simulink model "Arm_core_design_block"  (R2021a)
settings: Solver=VariableStepAuto  StartTime=0.0  StopTime=500  RelTol=1e-3
undefined symbols (not defined in the file or in its folder): AXI4, Lite
libraries: hdlBasic x907, xbsIndex_r4 x1
(part 7 of 7)

== system Arm_core_design_block/rotation9/Subsystem9 ==
  rst : Inport
  reg_i : Inport  Port=2
  Absolute1 : hdlBasic/Absolute  precision=User Defined  arith_type="Signed  (2's comp)"  n_bits=16  bin_pt=13  quantization=Truncate  overflow=Saturate  en=off  latency=0  XmcBlockStatus=1  maskContainerNames=tabcontainer1  block_type=abs  block_config=sysgen:Abs_config
  Accumulator1 : hdlBasic/Accumulator  operation=Add  n_bits=16  overflow=Wrap  scale=1  rst=on  hasbypass=off  en=on  latency=1  msb_inp=100  msb=100  lsb=-100  use_behavioral_HDL=on  implementation=Fabric  XmcBlockStatus=1  maskContainerNames=group3  block_type=accum  block_config=sysgen:Accum_config
  Constant4 : hdlBasic/Constant  const=0.019  gui_display_data_type=Fixed-point  arith_type=Signed (2's comp)  n_bits=16  bin_pt=14  preci_type=Single  exp_width=8  frac_width=24  explicit_period=off  period=1  XmcBlockStatus=1  maskContainerNames=tabcontainer1  block_type=constant  block_config=sysgen:Constant_config
  Constant5 : hdlBasic/Constant  const=1  gui_display_data_type=Fixed-point  arith_type=Unsigned  n_bits=16  bin_pt=1  preci_type=Single  exp_width=8  frac_width=24  explicit_period=off  period=1  XmcBlockStatus=1  maskContainerNames=tabcontainer1  block_type=constant  block_config=sysgen:Constant_config
  Constant6 : hdlBasic/Constant  const=3  gui_display_data_type=Fixed-point  arith_type=Unsigned  n_bits=16  bin_pt=1  preci_type=Single  exp_width=8  frac_width=24  explicit_period=off  period=1  XmcBlockStatus=1  maskContainerNames=tabcontainer1  block_type=constant  block_config=sysgen:Constant_config
  Constant7 : hdlBasic/Constant  const=0  gui_display_data_type=Boolean  arith_type=Boolean  n_bits=16  bin_pt=1  preci_type=Single  exp_width=8  frac_width=24  explicit_period=off  period=1  XmcBlockStatus=1  maskContainerNames=tabcontainer1  block_type=constant  block_config=sysgen:Constant_config
  Mux1 : hdlBasic/Mux  inputs=2  en=off  latency=0  precision=Full  arith_type=Unsigned  n_bits=16  bin_pt=14  quantization=Truncate  overflow=Wrap  XmcBlockStatus=1  maskContainerNames=tabcontainer1  block_type=mux  block_config=sysgen:Mux_config
  Register1 : hdlBasic/Register  init=0  rst=on  en=on  XmcBlockStatus=1  maskContainerNames=tabcontainer1  block_type=register  block_config=sysgen:Register_config
  Relational2 : hdlBasic/Relational  mode=a>b  op_type=Bool  en=off  latency=0  XmcBlockStatus=1  maskContainerNames=tabcontainer1  block_type=relational  block_config=sysgen:Relational_config
  Relational3 : hdlBasic/Relational  mode=a>b  op_type=Bool  en=off  latency=0  XmcBlockStatus=1  maskContainerNames=tabcontainer1  block_type=relational  block_config=sysgen:Relational_config
  reg_o : Outport
  wires:
  Constant5/1 -> Accumulator1/1
  Relational2/1 -> Mux1/2
  Constant7/1 -> Mux1/3
  reg_i/1 -> Absolute1/1, Register1/1
  rst/1 -> Register1/2, Accumulator1/2
  Constant6/1 -> Relational3/2
  Accumulator1/1 -> Relational3/1
  Relational3/1 -> Mux1/1
  Mux1/1 -> Register1/3, Accumulator1/3
  Absolute1/1 -> Relational2/1
  Constant4/1 -> Relational2/2
  Register1/1 -> reg_o/1
